simulink model "controllo_LQ_integrale_LMI"  (R2021a)
settings: Solver=VariableStepAuto  StartTime=0.0  StopTime=tsim  RelTol=1e-3
values from neighbouring files (symbols this model uses):
  b = 20    [main.m]
  c = 718    [main.m]
  F_lmi_int_fb = F_lmi_int(:,1:nx)    [main.m]
  F_lmi_int_ff = F_lmi_int(:,nx+1)    [main.m]
  f_w = 0    [main.m]
  g = 9.81    [main.m]
  k = 2.5    [main.m]
  m = 500    [main.m]
  p_a = 1.184    [main.m]
  theta_a = 298    [main.m]
  u_eq = k*(theta - theta_a)    (= 199.411134904)    [main.m]
  V = 2000    [main.m]
  x_eq = [600;0;theta]    [main.m]
undefined symbols (not defined in the file or in its folder): Cd
settings Model: Creator=Randy  LastModifiedBy=Randy

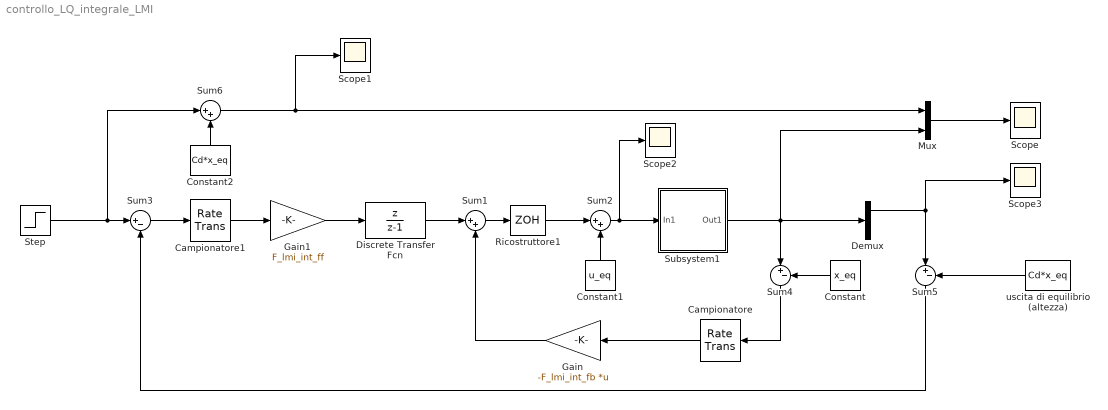
== system controllo_LQ_integrale_LMI ==
  Campionatore : RateTransition  OutPortSampleTime=Tc
  Campionatore1 : RateTransition  OutPortSampleTime=Tc
  Constant : Constant  Value=x_eq
  Constant1 : Constant  Value=u_eq
  Constant2 : Constant  Value=Cd*x_eq
  Demux : Demux  Outputs=nx
  Discrete Transfer Fcn : DiscreteTransferFcn  Numerator=[1 0]  Denominator=[1 -1]
  Gain : Gain  Gain=-F_lmi_int_fb  Multiplication=Matrix(K*u)
  Gain1 : Gain  Gain=F_lmi_int_ff
  Mux : Mux  Inputs=2
  Ricostruttore1 : ZeroOrderHold  SampleTime=-1
  Scope{,1..3} (4 alike) : Scope
  Step : Step  After=15  SampleTime=0
  Subsystem1 : Subsystem
  Sum1 : Sum  Inputs=|++
  Sum2 : Sum  Inputs=|++
  Sum3 : Sum  Inputs=|+-
  Sum4 : Sum  Inputs=|+-
  Sum5 : Sum  Inputs=|+-
  Sum6 : Sum  Inputs=|++
  uscita di equilibrio (altezza) : Constant  Value=Cd*x_eq  VectorParams1D=off
  wires:
  Constant/1 -> Sum4/2
  Campionatore/1 -> Gain/1
  Sum4/1 -> Campionatore/1
  Discrete Transfer Fcn/1 -> Sum1/1
  Gain/1 -> Sum1/2
  Sum1/1 -> Ricostruttore1/1
  Subsystem1/1(Out1) -> Mux/2, Demux/1, Sum4/1
  Ricostruttore1/1 -> Sum2/1
  Sum2/1 -> Scope2/1, Subsystem1/1(In1)
  Constant1/1 -> Sum2/2
  Gain1/1 -> Discrete Transfer Fcn/1
  Campionatore1/1 -> Gain1/1
  Sum3/1 -> Campionatore1/1
  Step/1 -> Sum6/1, Sum3/1
  Sum5/1 -> Sum3/2
  Sum6/1 -> Mux/1, Scope1/1
  Constant2/1 -> Sum6/2
  uscita di equilibrio (altezza)/1 -> Sum5/2
  Demux/1 -> Scope3/1, Sum5/1
  Mux/1 -> Scope/1

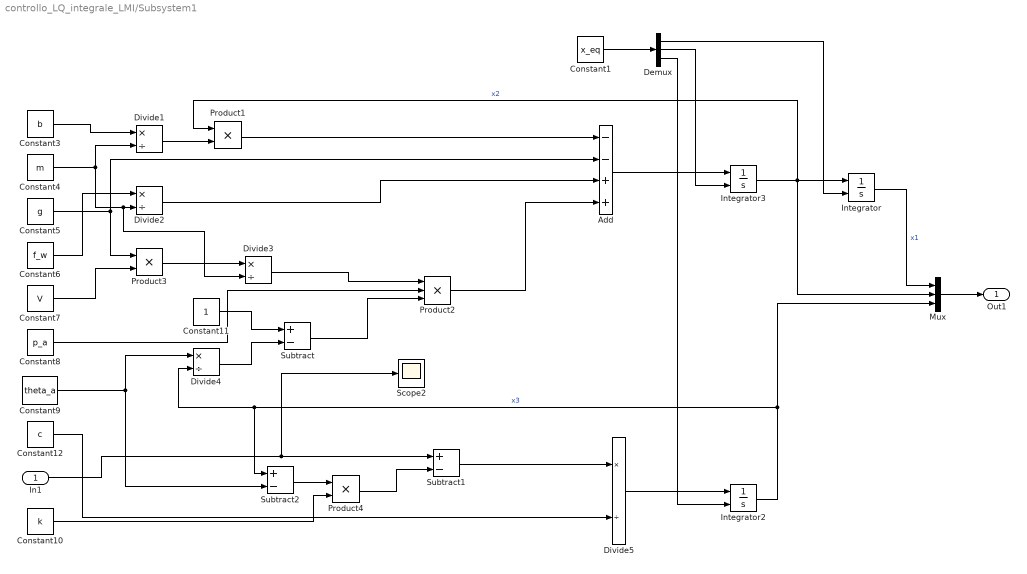
== system controllo_LQ_integrale_LMI/Subsystem1 ==
  In1 : Inport
  Add : Sum  Inputs=--++
  Constant1 : Constant  Value=x_eq
  Constant10 : Constant  Value=k
  Constant11 : Constant
  Constant12 : Constant  Value=c
  Constant3 : Constant  Value=b
  Constant4 : Constant  Value=m
  Constant5 : Constant  Value=g
  Constant6 : Constant  Value=f_w
  Constant7 : Constant  Value=V
  Constant8 : Constant  Value=p_a
  Constant9 : Constant  Value=theta_a
  Demux : Demux  Outputs=3
  Divide{1..5} (5 alike) : Product  Inputs=*/
  Integrator : Integrator  InitialConditionSource=external  InitialCondition=20
  Integrator2 : Integrator  InitialConditionSource=external  InitialCondition=200
  Integrator3 : Integrator  InitialConditionSource=external
  Mux : Mux  Inputs=3
  Product1 : Product
  Product2 : Product  Inputs=3
  Product3 : Product
  Product4 : Product
  Scope2 : Scope
  Subtract : Sum  Inputs=+-
  Subtract1 : Sum  Inputs=+-
  Subtract2 : Sum  Inputs=+-
  Out1 : Outport
  wires:
  Integrator2/1 -> Mux/3, Divide4/2, Subtract2/1  "x3"
  Subtract1/1 -> Divide5/1
  Constant6/1 -> Divide2/1
  Constant12/1 -> Divide5/2
  Divide5/1 -> Integrator2/1
  Constant8/1 -> Product2/2
  Add/1 -> Integrator3/1
  Mux/1 -> Out1/1
  Divide3/1 -> Product2/1
  Product1/1 -> Add/1
  Product3/1 -> Divide3/1
  Constant4/1 -> Divide1/2, Divide2/2, Divide3/2
  Integrator/1 -> Mux/1  "x1"
  Divide2/1 -> Add/3
  Integrator3/1 -> Mux/2, Integrator/1, Product1/1  "x2"
  Constant11/1 -> Subtract/1
  Product4/1 -> Subtract1/2
  Constant3/1 -> Divide1/1
  Divide1/1 -> Product1/2
  Subtract2/1 -> Product4/1
  Product2/1 -> Add/4
  Constant7/1 -> Product3/2
  Constant10/1 -> Product4/2
  Divide4/1 -> Subtract/2
  Constant5/1 -> Add/2, Product3/1
  Constant9/1 -> Divide4/1, Subtract2/2
  In1/1 -> Subtract1/1, Scope2/1
  Subtract/1 -> Product2/3
  Constant1/1 -> Demux/1
  Demux/2 -> Integrator3/2
  Demux/3 -> Integrator2/2
  Demux/1 -> Integrator/2
